simulink model "Variables_Estado_Red_Neuronal"  (R2016a)
settings: Solver=VariableStepAuto  StartTime=0.0  StopTime=100  RelTol=1e-3
undefined symbols (not defined in the file or in its folder): A, B
settings Model: Creator=Daniel  LastModifiedBy=Daniel

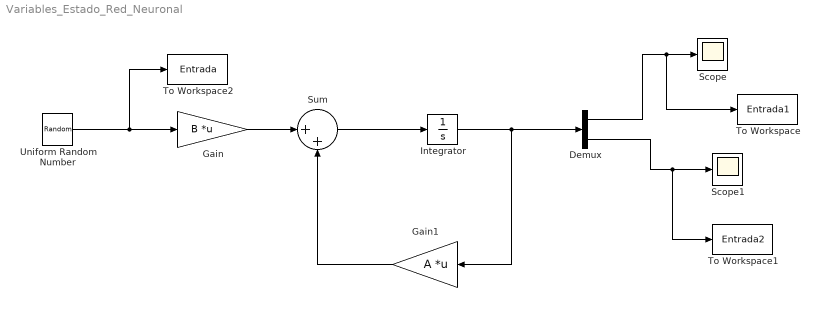
== system Variables_Estado_Red_Neuronal ==
  Demux : Demux  Outputs=2
  Gain : Gain  Gain=B  Multiplication=Matrix(K*u)
  Gain1 : Gain  Gain=A  Multiplication=Matrix(K*u)
  Integrator : Integrator
  Scope : Scope
  Scope1 : Scope
  Sum : Sum  Inputs=|++
  To Workspace : ToWorkspace  VariableName=Entrada1  SampleTime=0.1
  To Workspace1 : ToWorkspace  VariableName=Entrada2  SampleTime=0.1
  To Workspace2 : ToWorkspace  VariableName=Entrada  SampleTime=0.1
  Uniform Random Number : UniformRandomNumber  Minimum=0  Maximum=5  SampleTime=5
  wires:
  Uniform Random Number/1 -> To Workspace2/1, Gain/1
  Gain/1 -> Sum/1
  Gain1/1 -> Sum/2
  Sum/1 -> Integrator/1
  Integrator/1 -> Gain1/1, Demux/1
  Demux/2 -> To Workspace1/1, Scope1/1
  Demux/1 -> To Workspace/1, Scope/1
